simulink model "EcoSIM3_P2_C2_WIP"  (R2014b)
settings: Solver=ode1  SolverMode=SingleTasking  StartTime=0.0  StopTime=4  FixedStep=0.01  RelTol=1e-3
PostLoadFcn:
  | %, if any(exist('dsrtsu_mdlpostloadfcn', 'file') == [2, 3, 6]), try dsrtsu_mdlpostloadfcn('Execute', bdroot); catch fprintf('Error in PostLoadFcn (dsrtsu_mdlpostloadfcn) for model "%s":\n %s\n', bdroot, lasterr); end, end,
InitFcn:
  | tic
  | %Startup_EcoSIM
undefined symbols (not defined in the file or in its folder): canChannel, Controls, DriveCycles, Driver, EM_EFF_MAP, EM_PwrLoss_MAP, EngPwr, EngSpd, EngTrq, Glbl, Overwritten_Mode, Plants, Power, sigbuilder_block, Torque, Trialmap, Veh_Dynamics
libraries: simulink x135, canmsglib x113, fl_lib x104, canlib x89, nesl_utility x56, sdl_lib x29, dspsigops x6, dspswit3 x5, dspstat3 x2, commnoisgen2 x1, dspfdesign x1
(part 10 of 21)

== system EcoSIM3_P2_C2_WIP/Supervisory Controller/Supervisory_IO/VNT Vector/Electrical Rx ==
  Bus Creator : BusCreator  Inputs=7
  Bus Creator{1,4..6,9} (5 alike) : BusCreator  Inputs=2
  Bus Creator2 : BusCreator  Inputs=1
  Bus Creator3 : BusCreator  Inputs=7
  Bus Creator7 : BusCreator  Inputs=1
  Bus Selector : BusSelector  OutputSignals=From_SoftECU.GM_Electrical_Out.Drive_Mode,From_SoftECU.GM_Electrical_Out.PRNDL,From_SoftECU.GM_Electrical_Out.Alpha_Low,From_SoftECU.GM_Electrical_Out.Alpha_High,From_SoftECU.GM_Electrical_Out.Accessory_Wake,From_SoftECU.GM_Electrical_Out.PRNDL_1,From_SoftECU.GM_Electrical_Out.PRNDL_2,From_SoftECU.ESS_Electrical_Out.chga_ena
  Ground{,1..8} (9 alike) : Ground
  Electrical_Rx : Outport
  wires:
  [VNT_Electrical_FromGCM] -> Bus Creator1/1
  [VNT_Electrical_From_SoftECU] -> Bus Creator1/2  "From_SoftECU"
  Bus Creator1/1 -> Bus Selector/1
  Bus Selector/1 -> Bus Creator/1  "<Drive_Mode>"
  Bus Selector/2 -> Bus Creator/2  "<PRNDL>"
  Bus Selector/3 -> Bus Creator/3  "<Alpha_Low>"
  Bus Selector/4 -> Bus Creator/4  "<Alpha_High>"
  Bus Selector/5 -> Bus Creator/5  "<Accessory_Wake>"
  Bus Selector/8 -> Bus Creator2/1  "<chga_ena>"
  Bus Creator/1 -> Bus Creator3/3  "GM_Electrical_Out"
  Bus Creator2/1 -> Bus Creator3/4  "ESS_Electrical_Out"
  Bus Creator3/1 -> Electrical_Rx/1  "Electrical_Rx"
  Ground/1 -> Bus Creator4/1  "Dummy1"
  Ground1/1 -> Bus Creator4/2  "Dummy2"
  Bus Creator4/1 -> Bus Creator3/5  "BAS_Electrical_Out"
  Ground3/1 -> Bus Creator5/2  "Dummy2"
  Ground2/1 -> Bus Creator5/1  "Dummy1"
  Bus Creator5/1 -> Bus Creator3/2  "Clutch_Transmission_Electrical_Out"
  Ground5/1 -> Bus Creator6/2  "Dummy2"
  Ground4/1 -> Bus Creator6/1  "Dummy1"
  Bus Creator6/1 -> Bus Creator3/6  "ICE_Electrical_Out"
  Ground7/1 -> Bus Creator9/2  "Dummy2"
  Ground6/1 -> Bus Creator9/1  "Dummy1"
  Bus Creator9/1 -> Bus Creator3/1  "EM_Electrical_Out"
  Ground8/1 -> Bus Creator7/1  "<Dummy_Electrical1>"
  Bus Creator7/1 -> Bus Creator3/7  "CP1_Electrical_Out"
  Bus Selector/6 -> Bus Creator/6  "<PRNDL_1>"
  Bus Selector/7 -> Bus Creator/7  "<PRNDL_2>"

== system EcoSIM3_P2_C2_WIP/Supervisory Controller/Supervisory_IO/VNT Vector/Electrical Tx ==
  Electrical Tx : Inport
  Bus Creator : BusCreator  Inputs=2
  Bus Selector : BusSelector  OutputSignals=PON,chga_wake
  tag scope: VNT_Electrical_FromMABx=global
  wires:
  Bus Creator/1 -> [VNT_Electrical_FromMABx]  "Supervisory_Electrical_Out"
  Bus Selector/2 -> Bus Creator/2  "<chga_wake>"
  Bus Selector/1 -> Bus Creator/1  "<PON>"
  Electrical Tx/1 -> Bus Selector/1

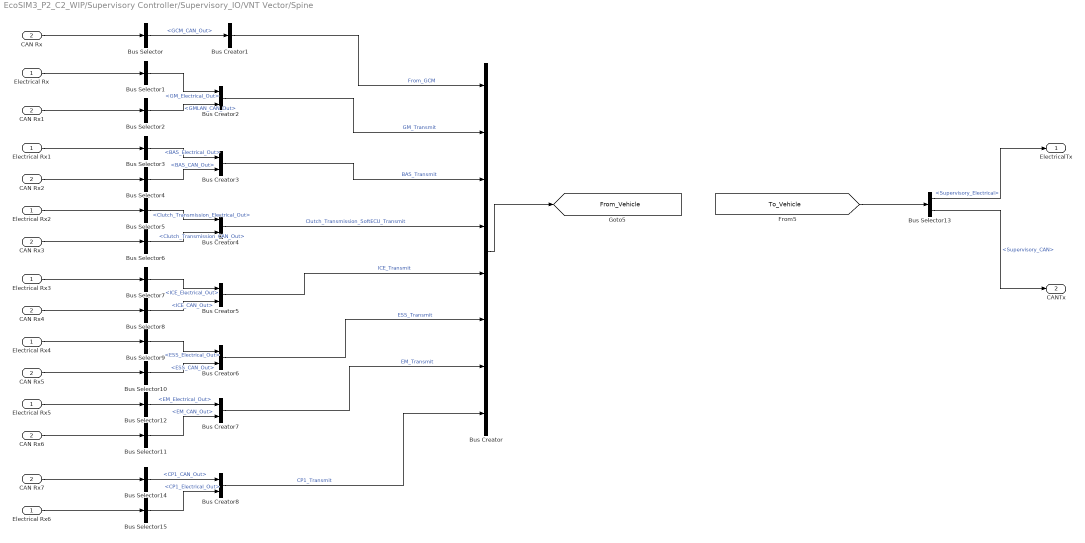
== system EcoSIM3_P2_C2_WIP/Supervisory Controller/Supervisory_IO/VNT Vector/Spine ==
  Electrical Rx : Inport
  CAN Rx : Inport  Port=2
  Bus Creator : BusCreator  Inputs=8
  Bus Creator1 : BusCreator  Inputs=1
  Bus Creator{2..8} (7 alike) : BusCreator  Inputs=2
  Bus Selector : BusSelector  OutputSignals=GCM_CAN_Out
  Bus Selector1 : BusSelector  OutputSignals=GM_Electrical_Out
  Bus Selector10 : BusSelector  OutputSignals=ESS_CAN_Out
  Bus Selector11 : BusSelector  OutputSignals=EM_CAN_Out
  Bus Selector12 : BusSelector  OutputSignals=EM_Electrical_Out
  Bus Selector13 : BusSelector  OutputSignals=Supervisory_Electrical,Supervisory_CAN
  Bus Selector14 : BusSelector  OutputSignals=CP1_CAN_Out
  Bus Selector15 : BusSelector  OutputSignals=CP1_Electrical_Out
  Bus Selector2 : BusSelector  OutputSignals=GMLAN_CAN_Out
  Bus Selector3 : BusSelector  OutputSignals=BAS_Electrical_Out
  Bus Selector4 : BusSelector  OutputSignals=BAS_CAN_Out
  Bus Selector5 : BusSelector  OutputSignals=Clutch_Transmission_Electrical_Out
  Bus Selector6 : BusSelector  OutputSignals=Clutch_Transmission_CAN_Out
  Bus Selector7 : BusSelector  OutputSignals=ICE_Electrical_Out
  Bus Selector8 : BusSelector  OutputSignals=ICE_CAN_Out
  Bus Selector9 : BusSelector  OutputSignals=ESS_Electrical_Out
  CAN Rx{1..7} (7 alike) : InportShadow  Port=2
  Electrical Rx{1..6} (6 alike) : InportShadow
  ElectricalTx : Outport
  CANTx : Outport  Port=2
  tag scope: From_Vehicle=global
  wires:
  [To_Vehicle] -> Bus Selector13/1
  Bus Creator/1 -> [From_Vehicle]
  CAN Rx/1 -> Bus Selector/1
  Electrical Rx/1 -> Bus Selector1/1
  Bus Selector/1 -> Bus Creator1/1  "<GCM_CAN_Out>"
  Bus Creator1/1 -> Bus Creator/1  "From_GCM"
  CAN Rx1/1 -> Bus Selector2/1
  Bus Selector1/1 -> Bus Creator2/1  "<GM_Electrical_Out>"
  Bus Selector2/1 -> Bus Creator2/2  "<GMLAN_CAN_Out>"
  Bus Creator2/1 -> Bus Creator/2  "GM_Transmit"
  Electrical Rx1/1 -> Bus Selector3/1
  CAN Rx2/1 -> Bus Selector4/1
  Bus Selector3/1 -> Bus Creator3/1  "<BAS_Electrical_Out>"
  Bus Selector4/1 -> Bus Creator3/2  "<BAS_CAN_Out>"
  Bus Creator3/1 -> Bus Creator/3  "BAS_Transmit"
  Electrical Rx2/1 -> Bus Selector5/1
  CAN Rx3/1 -> Bus Selector6/1
  Bus Selector5/1 -> Bus Creator4/1  "<Clutch_Transmission_Electrical_Out>"
  Bus Selector6/1 -> Bus Creator4/2  "<Clutch_Transmission_CAN_Out>"
  Bus Creator4/1 -> Bus Creator/4  "Clutch_Transmission_SoftECU_Transmit"
  Electrical Rx3/1 -> Bus Selector7/1
  CAN Rx4/1 -> Bus Selector8/1
  Bus Selector7/1 -> Bus Creator5/1  "<ICE_Electrical_Out>"
  Bus Selector8/1 -> Bus Creator5/2  "<ICE_CAN_Out>"
  Bus Creator5/1 -> Bus Creator/5  "ICE_Transmit"
  Electrical Rx4/1 -> Bus Selector9/1
  CAN Rx5/1 -> Bus Selector10/1
  Bus Selector9/1 -> Bus Creator6/1  "<ESS_Electrical_Out>"
  Bus Selector10/1 -> Bus Creator6/2  "<ESS_CAN_Out>"
  Bus Creator6/1 -> Bus Creator/6  "ESS_Transmit"
  Electrical Rx5/1 -> Bus Selector12/1
  CAN Rx6/1 -> Bus Selector11/1
  Bus Selector12/1 -> Bus Creator7/1  "<EM_Electrical_Out>"
  Bus Selector11/1 -> Bus Creator7/2  "<EM_CAN_Out>"
  Bus Creator7/1 -> Bus Creator/7  "EM_Transmit"
  Bus Selector13/1 -> ElectricalTx/1  "<Supervisory_Electrical>"
  Bus Selector13/2 -> CANTx/1  "<Supervisory_CAN>"
  CAN Rx7/1 -> Bus Selector14/1
  Electrical Rx6/1 -> Bus Selector15/1
  Bus Selector14/1 -> Bus Creator8/1  "<CP1_CAN_Out>"
  Bus Selector15/1 -> Bus Creator8/2  "<CP1_Electrical_Out>"
  Bus Creator8/1 -> Bus Creator/8  "CP1_Transmit"

== system EcoSIM3_P2_C2_WIP/Powertrain/Accessories Power Module/Component Power/The Corrupter/Enabled Subsystem ==
  In1 : Inport
  In2 : Inport  Port=2
  Enable : EnablePort
  Integrator : Integrator  InitialCondition=100
  Product5 : Product  Inputs=*/  RndMeth=Zero
  Out1 : Outport
  wires:
  Integrator/1 -> Out1/1
  In2/1 -> Product5/2
  In1/1 -> Product5/1
  Product5/1 -> Integrator/1

== system EcoSIM3_P2_C2_WIP/Powertrain/Accessories Power Module/Component Power/The Corrupter/Switch Logic ==
  NonCorrupted : Inport
  Corrupted : Inport  Port=2
  Logic : Inport  Port=3
  Switch : Switch  Criteria=u2 > Threshold
  Signal Out : Outport
  wires:
  Switch/1 -> Signal Out/1
  Logic/1 -> Switch/2
  NonCorrupted/1 -> Switch/3
  Corrupted/1 -> Switch/1

== system EcoSIM3_P2_C2_WIP/Powertrain/Accessories Power Module/Component Power/The Corrupter/Switch Logic1 ==
  F : Inport
  L : Inport  Port=2
  NF : Inport  Port=3
  Switch : Switch  Criteria=u2 ~= 0
  Out1 : Outport
  wires:
  L/1 -> Switch/2
  Switch/1 -> Out1/1
  NF/1 -> Switch/3
  F/1 -> Switch/1

== system EcoSIM3_P2_C2_WIP/Powertrain/BAS Motor/ Compnent Model/Sensors/Sensor lag ==
  i : Inport
  1st Order LPF of 1ms in Discrete Form : DiscreteTransferFcn  Numerator=[0.6321]  Denominator=[1 -0.3679]
  o : Outport
  wires:
  i/1 -> 1st Order LPF of 1ms in Discrete Form/1
  1st Order LPF of 1ms in Discrete Form/1 -> o/1

== system EcoSIM3_P2_C2_WIP/Powertrain/BAS Motor/ Compnent Model/Sensors/Sensor lag1 ==
  i : Inport
  1st Order LPF of 1ms in Discrete Form : DiscreteTransferFcn  Numerator=[0.6321]  Denominator=[1 -0.3679]
  o : Outport
  wires:
  1st Order LPF of 1ms in Discrete Form/1 -> o/1
  i/1 -> 1st Order LPF of 1ms in Discrete Form/1

== system EcoSIM3_P2_C2_WIP/Powertrain/BAS Motor/Soft ECU/Algorithm/EEPROM Parameters ==
  note: Need to change this to reflect max speed of the BAS
  Bus Creator : BusCreator  Inputs=2
  Motor_MaxSpeed : Constant  Value=Plants.ICE.Mdl.Plant.red_line_w*Plants.Belt.GR
  POST_Fault : Constant  Value=0
  EEPROM param : Outport
  wires:
  Motor_MaxSpeed/1 -> Bus Creator/1  "Motor_MaxSpeed"
  Bus Creator/1 -> EEPROM param/1
  POST_Fault/1 -> Bus Creator/2  "POST_Fault"

== system EcoSIM3_P2_C2_WIP/Powertrain/BAS Motor/Soft ECU/Algorithm/Faults ==
  Bus Creator : BusCreator  Inputs=3
  Fault_U : Constant  Value=0
  Fault_V : Constant  Value=0
  Fault_W : Constant  Value=0
  Logical Operator : Logic  Operator=OR  Inputs=3  AllPortsSameDT=off  OutDataTypeStr=boolean
  MotorFault : Outport
  CAN : Outport  Port=2
  wires:
  Fault_V/1 -> Logical Operator/2, Bus Creator/2  "Fault_V"
  Bus Creator/1 -> CAN/1
  Fault_U/1 -> Logical Operator/3, Bus Creator/1  "Fault_U"
  Fault_W/1 -> Logical Operator/1, Bus Creator/3  "Fault_W"
  Logical Operator/1 -> MotorFault/1  "MotorFault"

== system EcoSIM3_P2_C2_WIP/Powertrain/BAS Motor/Soft ECU/Algorithm/Torque Determination ==
  Speed : Inport
  IQ : Inport  Port=2
  Gain : Gain  Gain=9.54929659643
  Gain2 : Gain  Gain=9.54929659643
  Gain3 : Gain  Gain=-1
  Gain4 : Gain  Gain=-1
  Iq Lookup1 : Lookup_n-D  BreakpointsForDimension1=Plants.BAS.Mdl.Plant.Iq_reverse  BreakpointsForDimension2=Plants.BAS.Mdl.Plant.Rpm  Table=Plants.BAS.Mdl.Plant.Torque_Iq_1  InternalRulePriority=Speed  RndMeth=Simplest  InputSameDT=on
  Iq Lookup2 : Lookup_n-D  BreakpointsForDimension1=Plants.BAS.Mdl.Plant.Iq_reverse  BreakpointsForDimension2=Plants.BAS.Mdl.Plant.Rpm  Table=Plants.BAS.Mdl.Plant.Torque_Iq_1  InternalRulePriority=Speed  RndMeth=Simplest  InputSameDT=on
  Switch1 : Switch  Criteria=u2 > Threshold
  Switch2 : Switch  Criteria=u2 > Threshold
  Out1 : Outport
  wires:
  Gain2/1 -> Iq Lookup2/2
  Switch1/1 -> Iq Lookup1/1, Iq Lookup2/1
  Gain3/1 -> Switch1/3
  Iq Lookup2/1 -> Switch2/1
  Gain4/1 -> Switch2/3
  IQ/1 -> Switch1/1, Gain3/1, Switch1/2, Switch2/2
  Switch2/1 -> Out1/1
  Gain/1 -> Iq Lookup1/2
  Iq Lookup1/1 -> Gain4/1
  Speed/1 -> Gain2/1, Gain/1

== system EcoSIM3_P2_C2_WIP/Powertrain/Clutch_Transmission2/Trans_Plant/Plant/Gear1-2 ==
  In1 : Inport
  Bus Creator : BusCreator  Inputs=3
  Double-Sided Synchronizer : sdl_lib/Clutches/Double-Sided Synchronizer  model=1  max_torque=1000 N*m  n_teeth=6  clutch_backlash=10 deg  radius=200 mm  clutch_stiffness=1e+7 N*m/rad  clutch_damping=100 N*m/(rad/s)  fric_coeff=0.05  engagement_speed=Inf rad/s  d_o=150 mm  d_i=100 mm  theta=12 deg  friction_model=1  mu_coulomb=0.7  mu_w_vector=[ 0 0.1 0.2 0.3 0.4 0.5 1 2 5 10 100 1000 ] rad/s  mu_coulomb_vector=[ 0.29 0.28 0.26 0.22 0.21 0.2 0.2 0.19 0.19 0.19 0.19 0.19 ]  mu_interp_method=1  mu_extrap_method=1  mu_static=0.9  w_tol=0.001 rad/s  force_min=1 N  peak_force=3 N  width=3 mm  detent_visc_fric_transl=0.1 N/(m/s)  friction_ratio=0.01  v_thr=0.05 m/s  dog_clutch_ring_hub_gap=5 mm  engagement_overlap=3 mm  tooth_height=10 mm  cone_clutch_ring_hub_gap=3 mm  dog_clutch_transl_stiffness=1e+6 N/m  cone_clutch_transl_stiffness=1e+6 N/m  dog_clutch_transl_damping=1000 N/(m/s)  cone_clutch_transl_damping=1000 N/(m/s)  dog_clutch_visc_fric_transl=100 N/(m/s)  initial_state_locked=3  dog_clutch_init_pos=0 mm  cone_clutch_init_pos=0 mm  init_rel_angle_A=0 deg  init_rel_angle_B=0 deg
  Gain : Gain  Gain=1000
  Gain1 : Gain  Gain=1000
  Ideal Force Source : fl_lib/Mechanical/Mechanical Sources/Ideal Force Source
  Mechanical Translational Reference : fl_lib/Mechanical/Translational Elements/Mechanical Translational Reference
  Memory : Memory
  PI : Subsystem
  PS-Simulink Converter : nesl_utility/PS-Simulink Converter  PhysicalDomain=network_engine_domain  SubClassName=ps_output  LeftPortType=input  RightPortType=output  PseudoPeriodic=off  Frequencies=[]  Unit=1  AffineConversion=off
  PS-Simulink Converter1 : nesl_utility/PS-Simulink Converter  PhysicalDomain=network_engine_domain  SubClassName=ps_output  LeftPortType=input  RightPortType=output  PseudoPeriodic=off  Frequencies=[]  Unit=1  AffineConversion=off
  Rate Transition2 : RateTransition
  Scope7 : Scope
      settings: SaveName=ScopeData7
  Shaft Position : Subsystem
  Shift linkage mass : fl_lib/Mechanical/Translational Elements/Mass  mass=1 kg  v_specify=on  v_priority=High  v=0 m/s  f_specify=off  f_priority=High  f=0 N
  Simple Gear : sdl_lib/Gears/Simple Gear  ratio=Plants.Trans.Mdl.Plant.GR(1)  rotation_direction=1  friction_model=1  T_noload=0.1 N*m  T_nom=5 N*m  efficiency_nom=0.8  efficiency=0.8  mu_visc=[ 0 0 ] N*m/(rad/s)  w_thr=0.01 rad/s
  Simple Gear1 : sdl_lib/Gears/Simple Gear  ratio=Plants.Trans.Mdl.Plant.GR(2)  rotation_direction=1  friction_model=1  T_noload=0.1 N*m  T_nom=5 N*m  efficiency_nom=0.8  efficiency=0.8  mu_visc=[ 0 0 ] N*m/(rad/s)  w_thr=0.01 rad/s
  Simulink-PS Converter : nesl_utility/Simulink-PS Converter  PhysicalDomain=network_engine_domain  SubClassName=ps_input  LeftPortType=input  RightPortType=output  PseudoPeriodic=off  Frequencies=[]  NoiseDistribution=none  NoiseParameters=[]  Unit=N  AffineConversion=off  InputFiltering=on  SimscapeFilterOrder=1  InputFilterTimeConstant=0.01  UdotUserProvided=1
  Out : PMIOPort  Port=1  Side=Right
  In : PMIOPort  Port=2  Side=Left
  ShaftPosn : Outport
  wires:
  Rate Transition2/1 -> Simulink-PS Converter/1, Scope7/1
  PI/1(Force) -> Rate Transition2/1
  PS-Simulink Converter/1 -> Gain/1
  PS-Simulink Converter1/1 -> Gain1/1
  Gain/1 -> Memory/1, Shaft Position/1(Position_mm), Bus Creator/2  "Shaft_1-2_Dog_Clutch_posn_mm"
  Memory/1 -> PI/1(Actual_Pos)
  Gain1/1 -> Bus Creator/3  "Shaft_1-2_Cone_Clutch_posn_mm"
  In1/1 -> PI/2(Desired_Pos)
  Bus Creator/1 -> ShaftPosn/1  "Shaft_1-2"
  Shaft Position/1(Position) -> Bus Creator/1  "Shaft_1-2_Position"
  connections:
  Ideal Force Source/LConn1 -- Double-Sided Synchronizer/LConn1 -- Shift linkage mass/LConn1
  Ideal Force Source/RConn2 -- Mechanical Translational Reference/LConn1
  Ideal Force Source/RConn1 -- Simulink-PS Converter/RConn1
  Double-Sided Synchronizer/LConn3 -- Simple Gear/RConn1
  Double-Sided Synchronizer/RConn3 -- Simple Gear1/RConn1
  PS-Simulink Converter/LConn1 -- Double-Sided Synchronizer/RConn1
  Double-Sided Synchronizer/RConn2 -- PS-Simulink Converter1/LConn1
  Out/RConn1 -- Double-Sided Synchronizer/LConn2
  In/RConn1 -- Simple Gear/LConn1 -- Simple Gear1/LConn1

== system EcoSIM3_P2_C2_WIP/Powertrain/Clutch_Transmission2/Trans_Plant/Plant/Gear3-4 ==
  In1 : Inport
  Bus Creator : BusCreator  Inputs=3
  Double-Sided Synchronizer : sdl_lib/Clutches/Double-Sided Synchronizer  model=1  max_torque=1000 N*m  n_teeth=6  clutch_backlash=10 deg  radius=200 mm  clutch_stiffness=1e+7 N*m/rad  clutch_damping=100 N*m/(rad/s)  fric_coeff=0.05  engagement_speed=Inf rad/s  d_o=150 mm  d_i=100 mm  theta=12 deg  friction_model=1  mu_coulomb=0.7  mu_w_vector=[ 0 0.1 0.2 0.3 0.4 0.5 1 2 5 10 100 1000 ] rad/s  mu_coulomb_vector=[ 0.29 0.28 0.26 0.22 0.21 0.2 0.2 0.19 0.19 0.19 0.19 0.19 ]  mu_interp_method=1  mu_extrap_method=1  mu_static=0.9  w_tol=0.001 rad/s  force_min=1 N  peak_force=3 N  width=3 mm  detent_visc_fric_transl=0.1 N/(m/s)  friction_ratio=0.01  v_thr=0.05 m/s  dog_clutch_ring_hub_gap=5 mm  engagement_overlap=3 mm  tooth_height=10 mm  cone_clutch_ring_hub_gap=3 mm  dog_clutch_transl_stiffness=1e+6 N/m  cone_clutch_transl_stiffness=1e+6 N/m  dog_clutch_transl_damping=1000 N/(m/s)  cone_clutch_transl_damping=1000 N/(m/s)  dog_clutch_visc_fric_transl=100 N/(m/s)  initial_state_locked=3  dog_clutch_init_pos=0 mm  cone_clutch_init_pos=0 mm  init_rel_angle_A=0 deg  init_rel_angle_B=0 deg
  Gain : Gain  Gain=1000
  Gain1 : Gain  Gain=1000
  Ideal Force Source : fl_lib/Mechanical/Mechanical Sources/Ideal Force Source
  Mechanical Translational Reference : fl_lib/Mechanical/Translational Elements/Mechanical Translational Reference
  Memory : Memory
  PI2 : Subsystem
  PS-Simulink Converter : nesl_utility/PS-Simulink Converter  PhysicalDomain=network_engine_domain  SubClassName=ps_output  LeftPortType=input  RightPortType=output  PseudoPeriodic=off  Frequencies=[]  Unit=1  AffineConversion=off
  PS-Simulink Converter1 : nesl_utility/PS-Simulink Converter  PhysicalDomain=network_engine_domain  SubClassName=ps_output  LeftPortType=input  RightPortType=output  PseudoPeriodic=off  Frequencies=[]  Unit=1  AffineConversion=off
  Rate Transition2 : RateTransition
  Scope7 : Scope
      settings: SaveName=ScopeData7
  Shaft Position : Subsystem
  Shift linkage mass : fl_lib/Mechanical/Translational Elements/Mass  mass=1 kg  v_specify=on  v_priority=High  v=0 m/s  f_specify=off  f_priority=High  f=0 N
  Simple Gear2 : sdl_lib/Gears/Simple Gear  ratio=Plants.Trans.Mdl.Plant.GR(3)  rotation_direction=1  friction_model=1  T_noload=0.1 N*m  T_nom=5 N*m  efficiency_nom=0.8  efficiency=0.8  mu_visc=[ 0 0 ] N*m/(rad/s)  w_thr=0.01 rad/s
  Simple Gear3 : sdl_lib/Gears/Simple Gear  ratio=Plants.Trans.Mdl.Plant.GR(4)  rotation_direction=1  friction_model=1  T_noload=0.1 N*m  T_nom=5 N*m  efficiency_nom=0.8  efficiency=0.8  mu_visc=[ 0 0 ] N*m/(rad/s)  w_thr=0.01 rad/s
  Simulink-PS Converter : nesl_utility/Simulink-PS Converter  PhysicalDomain=network_engine_domain  SubClassName=ps_input  LeftPortType=input  RightPortType=output  PseudoPeriodic=off  Frequencies=[]  NoiseDistribution=none  NoiseParameters=[]  Unit=N  AffineConversion=off  InputFiltering=on  SimscapeFilterOrder=1  InputFilterTimeConstant=0.01  UdotUserProvided=1
  Out : PMIOPort  Port=1  Side=Right
  In : PMIOPort  Port=2  Side=Left
  ShaftPosn : Outport
  wires:
  Gain1/1 -> Bus Creator/3  "Shaft_3-4_Cone_Clutch_posn_mm"
  Gain/1 -> Bus Creator/2, Memory/1, Shaft Position/1(Position_mm)  "Shaft_3-4_Dog_Clutch_posn_mm"
  PS-Simulink Converter1/1 -> Gain1/1
  PS-Simulink Converter/1 -> Gain/1
  PI2/1(Force) -> Rate Transition2/1
  Rate Transition2/1 -> Scope7/1, Simulink-PS Converter/1
  Bus Creator/1 -> ShaftPosn/1  "Shaft_3-4"
  Memory/1 -> PI2/1(Actual_Pos)
  In1/1 -> PI2/2(Desired_Pos)
  Shaft Position/1(Position) -> Bus Creator/1  "Shaft_3-4_Position"
  connections:
  Out/RConn1 -- Double-Sided Synchronizer/LConn2
  Double-Sided Synchronizer/RConn2 -- PS-Simulink Converter1/LConn1
  PS-Simulink Converter/LConn1 -- Double-Sided Synchronizer/RConn1
  Simple Gear3/RConn1 -- Double-Sided Synchronizer/RConn3
  Simple Gear2/RConn1 -- Double-Sided Synchronizer/LConn3
  Ideal Force Source/RConn1 -- Simulink-PS Converter/RConn1
  Ideal Force Source/RConn2 -- Mechanical Translational Reference/LConn1
  Double-Sided Synchronizer/LConn1 -- Shift linkage mass/LConn1 -- Ideal Force Source/LConn1
  Simple Gear2/LConn1 -- In/RConn1 -- Simple Gear3/LConn1

== system EcoSIM3_P2_C2_WIP/Powertrain/Clutch_Transmission2/Trans_Plant/Plant/Gear5-R ==
  In1 : Inport
  Bus Creator : BusCreator  Inputs=3
  Double-Sided Synchronizer : sdl_lib/Clutches/Double-Sided Synchronizer  model=1  max_torque=1000 N*m  n_teeth=6  clutch_backlash=10 deg  radius=200 mm  clutch_stiffness=1e+7 N*m/rad  clutch_damping=100 N*m/(rad/s)  fric_coeff=0.05  engagement_speed=Inf rad/s  d_o=150 mm  d_i=100 mm  theta=12 deg  friction_model=1  mu_coulomb=0.7  mu_w_vector=[ 0 0.1 0.2 0.3 0.4 0.5 1 2 5 10 100 1000 ] rad/s  mu_coulomb_vector=[ 0.29 0.28 0.26 0.22 0.21 0.2 0.2 0.19 0.19 0.19 0.19 0.19 ]  mu_interp_method=1  mu_extrap_method=1  mu_static=0.9  w_tol=0.001 rad/s  force_min=1 N  peak_force=3 N  width=3 mm  detent_visc_fric_transl=0.1 N/(m/s)  friction_ratio=0.01  v_thr=0.05 m/s  dog_clutch_ring_hub_gap=5 mm  engagement_overlap=3 mm  tooth_height=10 mm  cone_clutch_ring_hub_gap=3 mm  dog_clutch_transl_stiffness=1e+6 N/m  cone_clutch_transl_stiffness=1e+6 N/m  dog_clutch_transl_damping=1000 N/(m/s)  cone_clutch_transl_damping=1000 N/(m/s)  dog_clutch_visc_fric_transl=100 N/(m/s)  initial_state_locked=3  dog_clutch_init_pos=0 mm  cone_clutch_init_pos=0 mm  init_rel_angle_A=0 deg  init_rel_angle_B=0 deg
  Gain : Gain  Gain=1000
  Gain1 : Gain  Gain=1000
  Ideal Force Source : fl_lib/Mechanical/Mechanical Sources/Ideal Force Source
  Mechanical Translational Reference : fl_lib/Mechanical/Translational Elements/Mechanical Translational Reference
  Memory : Memory
  PI2 : Subsystem
  PS-Simulink Converter : nesl_utility/PS-Simulink Converter  PhysicalDomain=network_engine_domain  SubClassName=ps_output  LeftPortType=input  RightPortType=output  PseudoPeriodic=off  Frequencies=[]  Unit=1  AffineConversion=off
  PS-Simulink Converter1 : nesl_utility/PS-Simulink Converter  PhysicalDomain=network_engine_domain  SubClassName=ps_output  LeftPortType=input  RightPortType=output  PseudoPeriodic=off  Frequencies=[]  Unit=1  AffineConversion=off
  Rate Transition2 : RateTransition
  Scope7 : Scope
      settings: SaveName=ScopeData7
  Shaft Position : Subsystem
  Shift linkage mass : fl_lib/Mechanical/Translational Elements/Mass  mass=1 kg  v_specify=on  v_priority=High  v=0 m/s  f_specify=off  f_priority=High  f=0 N
  Simple Gear2 : sdl_lib/Gears/Simple Gear  ratio=Plants.Trans.Mdl.Plant.GR(5)  rotation_direction=1  friction_model=1  T_noload=0.1 N*m  T_nom=5 N*m  efficiency_nom=0.8  efficiency=0.8  mu_visc=[ 0 0 ] N*m/(rad/s)  w_thr=0.01 rad/s
  Simple Gear3 : sdl_lib/Gears/Simple Gear  ratio=2.76  rotation_direction=2  friction_model=1  T_noload=0.1 N*m  T_nom=5 N*m  efficiency_nom=0.8  efficiency=0.8  mu_visc=[ 0 0 ] N*m/(rad/s)  w_thr=0.01 rad/s
  Simulink-PS Converter : nesl_utility/Simulink-PS Converter  PhysicalDomain=network_engine_domain  SubClassName=ps_input  LeftPortType=input  RightPortType=output  PseudoPeriodic=off  Frequencies=[]  NoiseDistribution=none  NoiseParameters=[]  Unit=N  AffineConversion=off  InputFiltering=on  SimscapeFilterOrder=1  InputFilterTimeConstant=0.01  UdotUserProvided=1
  Out : PMIOPort  Port=1  Side=Right
  In : PMIOPort  Port=2  Side=Left
  ShaftPosn : Outport
  wires:
  In1/1 -> PI2/2(Desired_Pos)
  Memory/1 -> PI2/1(Actual_Pos)
  Bus Creator/1 -> ShaftPosn/1  "Shaft_5-R"
  Rate Transition2/1 -> Simulink-PS Converter/1, Scope7/1
  PI2/1(Force) -> Rate Transition2/1
  PS-Simulink Converter/1 -> Gain/1
  PS-Simulink Converter1/1 -> Gain1/1
  Gain/1 -> Bus Creator/2, Memory/1, Shaft Position/1(Position_mm)  "Shaft_5-R_Dog_Clutch_posn_mm"
  Gain1/1 -> Bus Creator/3  "Shaft_5-R_Cone_Clutch_posn_mm"
  Shaft Position/1(Position) -> Bus Creator/1  "Shaft_5-R_Position"
  connections:
  In/RConn1 -- Simple Gear2/LConn1 -- Simple Gear3/LConn1
  Ideal Force Source/LConn1 -- Shift linkage mass/LConn1 -- Double-Sided Synchronizer/LConn1
  Ideal Force Source/RConn2 -- Mechanical Translational Reference/LConn1
  Ideal Force Source/RConn1 -- Simulink-PS Converter/RConn1
  Simple Gear2/RConn1 -- Double-Sided Synchronizer/LConn3
  Simple Gear3/RConn1 -- Double-Sided Synchronizer/RConn3
  PS-Simulink Converter/LConn1 -- Double-Sided Synchronizer/RConn1
  Double-Sided Synchronizer/RConn2 -- PS-Simulink Converter1/LConn1
  Out/RConn1 -- Double-Sided Synchronizer/LConn2

== system EcoSIM3_P2_C2_WIP/Powertrain/Clutch_Transmission2/Trans_Plant/Plant/Subsystem ==
  In1 : Inport
  Bus Selector : BusSelector  OutputSignals=Shaft_1-2.Shaft_1-2_Position,Shaft_3-4.Shaft_3-4_Position,Shaft_5-R.Shaft_5-R_Position
  Determine Gear : Stateflow chart  Commented=on  TreatAsAtomicUnit=on
  Display : Display
  Gain : Gain
  Lookup Table based Gear : Subsystem  Commented=on
  Memory : Memory
  Mux : Mux  Inputs=3
  Scope : Scope
      settings: SaveName=ScopeData3
  Switch : Switch  Criteria=u2 > Threshold  Threshold=6
  Truth Table : Truth Table  TreatAsAtomicUnit=on
  Out1 : Outport
  tag scope: Shaft_Positions=global
  wires:
  In1/1 -> Bus Selector/1
  Bus Selector/3 -> Truth Table/3(u3), Mux/3  "<Shaft_5-R_Position>"
  Bus Selector/2 -> Truth Table/2(u2), Mux/2  "<Shaft_3-4_Position>"
  Bus Selector/1 -> Truth Table/1(u1), Mux/1  "<Shaft_1-2_Position>"
  Switch/1 -> Memory/1, Gain/1  "Mastershift_Gear"
  Gain/1 -> Display/1, Out1/1
  Mux/1 -> [Shaft_Positions], Scope/1
  Truth Table/1(y) -> Switch/3, Switch/2  "Mastershift_Gear"
  Memory/1 -> Switch/1

== system EcoSIM3_P2_C2_WIP/Powertrain/Electric Motor / Component Model/Plant/EM_Thermal_Model ==
  note: Instead of a heat source, add convection to the water
  note: A hotspot that will be the thermally weakest point
  note: Assume coolant out temp is same as motor temp
  EM_Power_Loss : Inport
  Conductive Heat Transfer : fl_lib/Thermal/Thermal Elements/Conductive Heat Transfer  area=4 cm^2  thickness=0.1 cm  th_cond=401 W/(m*K)  Q_specify=off  Q_priority=High  Q=0 J/s  T_specify=off  T_priority=High  T=0 K
  Constant1 : Constant  Value=293
  Convection to air : fl_lib/Thermal/Thermal Elements/Convective Heat Transfer  area=1111 cm^2  heat_tr_coeff=10 W/(m^2 * K)  Q_specify=off  Q_priority=High  Q=0 J/s  T_specify=off  T_priority=High  T=0 K
  EM_Over_Temp_Fault : Subsystem
  Gain : Gain  Gain=0.05
  Gain1 : Gain  Gain=0.95
  Heat Dissipated through coolant : Subsystem
  Heat absorbed by coolant : fl_lib/Thermal/Thermal Sources/Ideal Heat Flow Source
  Hotspot Heat : fl_lib/Thermal/Thermal Sources/Ideal Heat Flow Source
  Hotspot Thermal mass : fl_lib/Thermal/Thermal Elements/Thermal Mass  mass=0.1 kg  sp_heat=447 J/kg/K  Q_specify=off  Q_priority=High  Q=0 J/s  T_specify=off  T_priority=High  T=300 K
  Hotspot temp in °C : Scope
      settings: SaveName=ScopeData2
  Ideal Temperature Source : fl_lib/Thermal/Thermal Sources/Ideal Temperature Source
  Memory : Memory  X0=293
  Memory1 : Memory  X0=25
  Motor Heat Loss : fl_lib/Thermal/Thermal Sources/Ideal Heat Flow Source
  Motor Thermal Mass : fl_lib/Thermal/Thermal Elements/Thermal Mass  mass=35 kg  sp_heat=447 J/kg/K  Q_specify=off  Q_priority=High  Q=0 J/s  T_specify=off  T_priority=High  T=300 K
  Simulink-PS Converter : nesl_utility/Simulink-PS Converter  PhysicalDomain=network_engine_domain  SubClassName=ps_input  LeftPortType=input  RightPortType=output  PseudoPeriodic=off  Frequencies=[]  NoiseDistribution=none  NoiseParameters=[]  Unit=J/s  AffineConversion=off  InputFiltering=off  SimscapeFilterOrder=1  InputFilterTimeConstant=0.001  UdotUserProvided=1
  Simulink-PS Converter1 : nesl_utility/Simulink-PS Converter  PhysicalDomain=network_engine_domain  SubClassName=ps_input  LeftPortType=input  RightPortType=output  PseudoPeriodic=off  Frequencies=[]  NoiseDistribution=none  NoiseParameters=[]  Unit=J/s  AffineConversion=off  InputFiltering=off  SimscapeFilterOrder=1  InputFilterTimeConstant=0.001  UdotUserProvided=1
  Simulink-PS Converter2 : nesl_utility/Simulink-PS Converter  PhysicalDomain=network_engine_domain  SubClassName=ps_input  LeftPortType=input  RightPortType=output  PseudoPeriodic=off  Frequencies=[]  NoiseDistribution=none  NoiseParameters=[]  Unit=K  AffineConversion=off  InputFiltering=off  SimscapeFilterOrder=1  InputFilterTimeConstant=0.001  UdotUserProvided=1
  Solver Configuration : nesl_utility/Solver Configuration  PhysicalDomain=network_engine_domain  SubClassName=solver  LeftPortType=input  RightPortType=generic  Accelerate=off  Tones=[]  Harmonics=[]  SimulateNoise=off  Profile=off  UseLocalSampling=off  EnableSwitchedLinearOptims=on  FrequencyDomain=off  UseCCode=off  RelTol=0.001  AbsTol=1e-06  MinStep=1e-09  ToWorkspace=off  DoDC=off  ResidualTolerance=1e-09  UseLocalSolver=on  LocalSolverChoice=NE_BACKWARD_EULER_ADVANCER  LocalSolverSampleTime=0.01  DoFixedCost=off  MaxNonlinIter=3  MaxModeIter=2  LinearAlgebra=Sparse  DelaysMemoryBudget=1024  AutomaticFiltering=on  FilteringTimeConstant=0.001
  Temp Hotspot : Subsystem
  Temp Motor : Subsystem
  Thermal Reference{,2..4} (4 alike) : fl_lib/Thermal/Thermal Elements/Thermal Reference
  Out1 : Outport
  wires:
  Constant1/1 -> Simulink-PS Converter2/1
  Temp Hotspot/1(Temp C) -> Hotspot temp in °C/1  "EM_hotspot_Temperature_degC"
  Temp Motor/1(Temp K) -> Memory/1
  EM_Over_Temp_Fault/1(Out1) -> Out1/1  "EM_Temperature_degC"
  Memory/1 -> Heat Dissipated through coolant/1(Coolant Out Temp)
  EM_Power_Loss/1 -> Gain/1, Gain1/1  "EM_Power_loss_W"
  Gain/1 -> Simulink-PS Converter/1
  Gain1/1 -> Simulink-PS Converter1/1
  Temp Motor/2(Temp C) -> Memory1/1  "EM_Temperature_degC"
  Memory1/1 -> EM_Over_Temp_Fault/1(In1)  "EM_Temperature_degC"
  connections:
  Simulink-PS Converter2/RConn1 -- Ideal Temperature Source/RConn1
  Heat Dissipated through coolant/RConn1 -- Heat absorbed by coolant/RConn1
  Convection to air/RConn1 -- Ideal Temperature Source/LConn1
  Thermal Reference4/LConn1 -- Hotspot Heat/RConn2
  Simulink-PS Converter1/RConn1 -- Hotspot Heat/RConn1
  Thermal Reference/LConn1 -- Motor Heat Loss/RConn2
  Thermal Reference2/LConn1 -- Ideal Temperature Source/RConn2
  Thermal Reference3/LConn1 -- Heat absorbed by coolant/RConn2
  Motor Heat Loss/RConn1 -- Simulink-PS Converter/RConn1 -- Solver Configuration/RConn1
  Convection to air/LConn1 -- Temp Motor/LConn1 -- Conductive Heat Transfer/RConn1 -- Motor Thermal Mass/LConn1 -- Heat absorbed by coolant/LConn1 -- Motor Heat Loss/LConn1
  Conductive Heat Transfer/LConn1 -- Hotspot Thermal mass/LConn1 -- Temp Hotspot/LConn1 -- Hotspot Heat/LConn1

== system EcoSIM3_P2_C2_WIP/Powertrain/Electric Motor / Component Model/Sensors/Fault Insertation ==
  In1 : Inport
  Additional_Torque_Nm_Default : Constant  Value=0
  Gain : Gain  Gain=.3
  Ideal Torque Source1 : fl_lib/Mechanical/Mechanical Sources/Ideal Torque Source
  Mechanical Rotational Reference2 : fl_lib/Mechanical/Rotational Elements/Mechanical Rotational Reference
  OverTorque_Trigger : Switch  Criteria=u2 > Threshold  Threshold=0.5
  Simulink-PS Converter1 : nesl_utility/Simulink-PS Converter  PhysicalDomain=network_engine_domain  SubClassName=ps_input  LeftPortType=input  RightPortType=output  PseudoPeriodic=off  Frequencies=[]  NoiseDistribution=none  NoiseParameters=[]  Unit=1  AffineConversion=off  InputFiltering=off  SimscapeFilterOrder=1  InputFilterTimeConstant=0.001  UdotUserProvided=1
  Conn1 : PMIOPort  Port=1  Side=Right
  wires:
  [EM_OverTorque_Trigger] -> OverTorque_Trigger/2
  Additional_Torque_Nm_Default/1 -> OverTorque_Trigger/3
  OverTorque_Trigger/1 -> Simulink-PS Converter1/1
  In1/1 -> Gain/1
  Gain/1 -> OverTorque_Trigger/1
  connections:
  Simulink-PS Converter1/RConn1 -- Ideal Torque Source1/RConn1
  Ideal Torque Source1/RConn2 -- Mechanical Rotational Reference2/LConn1
  Ideal Torque Source1/LConn1 -- Conn1/RConn1

== system EcoSIM3_P2_C2_WIP/Powertrain/Electric Motor / Component Model/Sensors/Sensor lag ==
  i : Inport
  1st Order LPF of 1ms in Discrete Form : DiscreteTransferFcn  Numerator=[0.6321]  Denominator=[1 -0.3679]
  o : Outport
  wires:
  i/1 -> 1st Order LPF of 1ms in Discrete Form/1
  1st Order LPF of 1ms in Discrete Form/1 -> o/1

== system EcoSIM3_P2_C2_WIP/Powertrain/Electric Motor / Component Model/Sensors/Sensor lag1 ==
  i : Inport
  1st Order LPF of 1ms in Discrete Form : DiscreteTransferFcn  Numerator=[0.6321]  Denominator=[1 -0.3679]
  o : Outport
  wires:
  i/1 -> 1st Order LPF of 1ms in Discrete Form/1
  1st Order LPF of 1ms in Discrete Form/1 -> o/1

== system EcoSIM3_P2_C2_WIP/Powertrain/Electric Motor / Component Model/Sensors/Sensors ==
  note: Sensor Model: Place where we add Corrupter
  Bus Creator : BusCreator  Inputs=2
  Ideal Rotational Motion Sensor : fl_lib/Mechanical/Mechanical Sensors/Ideal Rotational Motion Sensor  offset=0 rad
  Ideal Torque Sensor : fl_lib/Mechanical/Mechanical Sensors/Ideal Torque Sensor
  Mechanical Rotational Reference1 : fl_lib/Mechanical/Rotational Elements/Mechanical Rotational Reference
  PS-Simulink Converter : nesl_utility/PS-Simulink Converter  PhysicalDomain=network_engine_domain  SubClassName=ps_output  LeftPortType=input  RightPortType=output  PseudoPeriodic=off  Frequencies=[]  Unit=1  AffineConversion=off
  PS-Simulink Converter1 : nesl_utility/PS-Simulink Converter  PhysicalDomain=network_engine_domain  SubClassName=ps_output  LeftPortType=input  RightPortType=output  PseudoPeriodic=off  Frequencies=[]  Unit=1  AffineConversion=off
  Sensor lag : Subsystem
  Sensor lag1 : Subsystem
  Shaft : PMIOPort  Port=1  Side=Left
  To_Plants : PMIOPort  Port=2  Side=Right
  EM_Shaft_out : Outport
  wires:
  Sensor lag/1(o) -> Bus Creator/1  "EM_Speed_produced_rad_per_s"
  Sensor lag1/1(o) -> Bus Creator/2  "EM_Torque_Produced_Nm"
  Bus Creator/1 -> EM_Shaft_out/1  "EM_Shaft"
  PS-Simulink Converter/1 -> Sensor lag/1(i)  "EM_Speed_produced_rad_per_s"
  PS-Simulink Converter1/1 -> Sensor lag1/1(i)  "EM_Torque_Produced_Nm"
  connections:
  Ideal Torque Sensor/LConn1 -- Shaft/RConn1 -- Ideal Rotational Motion Sensor/LConn1
  Ideal Rotational Motion Sensor/RConn1 -- Mechanical Rotational Reference1/LConn1
  PS-Simulink Converter/LConn1 -- Ideal Rotational Motion Sensor/RConn2
  PS-Simulink Converter1/LConn1 -- Ideal Torque Sensor/RConn2
  Ideal Torque Sensor/RConn1 -- To_Plants/RConn1

== system EcoSIM3_P2_C2_WIP/Powertrain/Electric Motor /Soft ECU/Algorithm/Normal Operation ==
  note: These signals are supposed to be
      |  coming in through CAN
  SignalIn : Inport
  FaultTrigger : Inport  Port=2
  Enable : EnablePort  StatesWhenEnabling=reset
  Bus Creator : BusCreator  Inputs=3
  Bus Selector : BusSelector  OutputSignals=Motor_MaxSpeed
  Bus Selector1 : BusSelector  OutputSignals=EM_Sensors.Motor_Speed,EM_Sensors.InternalMotorError,EM_CAN_Messages.EM_CAN.M192_Command_Message.Rotation_Direction,EM_CAN_Messages.EM_CAN.M192_Command_Message.Torque_Command,ESS_CAN_Out.BCM_Status.bcm_mainc_stat,EM_CAN_Messages.EM_CAN.M192_Command_Message.Inverter_Enable,EM_CAN_Messages.EM_Electrical.EM_Powerup
  Bus Selector4 : BusSelector  OutputSignals=EM_torque_cmd_value,EM_torque_cmd_trigger
  EEPROM Parameters1 : Subsystem
  Normal_Operation : Stateflow chart  TreatAsAtomicUnit=on
  Scope : Scope
      settings: SaveName=ScopeData58
  Switch : Switch  Criteria=u2 > Threshold  Threshold=0.5
  Status : Outport
  wires:
  Bus Selector1/3 -> Normal_Operation/3(Rotation_Direction)  "<Rotation_Direction>"
  Bus Selector1/4 -> Normal_Operation/4(Torque_Command)  "<Torque_Command>"
  SignalIn/1 -> Bus Selector1/1
  Bus Selector/1 -> Normal_Operation/8(Motor_MaxSpeed)  "<Motor_MaxSpeed>"
  Normal_Operation/1(Commanded_Torque) -> Switch/3
  EEPROM Parameters1/1(EEPROM param) -> Bus Selector/1
  Bus Selector1/5 -> Normal_Operation/5(batt_mainc_stat)  "<bcm_mainc_stat>"
  Bus Selector1/6 -> Normal_Operation/6(Inverter_Enable)  "<Inverter_Enable>"
  Switch/1 -> Scope/1, Bus Creator/1  "Commanded_Torque"
  FaultTrigger/1 -> Bus Selector4/1
  Bus Selector4/2 -> Switch/2  "<EM_torque_cmd_trigger>"
  Bus Selector4/1 -> Switch/1  "<EM_torque_cmd_value>"
  Bus Selector1/1 -> Normal_Operation/1(Motor_Speed)  "<Motor_Speed>"
  Bus Selector1/2 -> Normal_Operation/2(InternalMotorError)  "<InternalMotorError>"
  Bus Creator/1 -> Status/1  "RunningStatus"
  Normal_Operation/2(RUN_Fault) -> Bus Creator/2  "RUN_Fault"
  Normal_Operation/3(ShutdownRequest) -> Bus Creator/3  "ShutdownRequest"
  Bus Selector1/7 -> Normal_Operation/7(Power_up)  "<EM_Powerup>"

== system EcoSIM3_P2_C2_WIP/Powertrain/Electric Motor /Soft ECU/Algorithm/Rinehart Documentation ==

== system EcoSIM3_P2_C2_WIP/Powertrain/Electric Motor /Soft ECU/Algorithm/Startup_Shutdown ==
  SignalIn : Inport
  Faults : Inport  Port=2
  Bus Creator : BusCreator  Inputs=7
  Bus Selector : BusSelector  OutputSignals=EM_Sensors.EM_Temperature_degC,EM_Sensors.Motor_Speed,EM_Sensors.EM_Torque_Out_Nm,EM_CAN_Messages.EM_CAN.M192_Command_Message.Rotation_Direction,EM_CAN_Messages.EM_Electrical.EM_Powerup,EM_Sensors.InternalMotorError,ESS_CAN_Out.BCM_Status.bcm_mainc_stat,EM_CAN_Messages.EM_CAN.M192_Command_Message.Inverter_Enable
  Bus Selector1 : BusSelector  OutputSignals=KeySwMode,POST_Fault
  Bus Selector3 : BusSelector  OutputSignals=RUN_Fault,ShutdownRequest
  EEPROM Parameters : Subsystem
  Memory : Memory
  Memory1 : Memory
  Memory2 : Memory
  Startup-Shutdown : Stateflow chart  TreatAsAtomicUnit=on
  Subsystem : Subsystem
  Temperature Values Dummy : Subsystem
  Terminator : Terminator
  Inverter_Status : Outport
  VSM : Outport  Port=2
  wires:
  Startup-Shutdown/2(Inverter_Enable_Lockout) -> Bus Creator/6  "Inverter_Enable_Lockout"
  Bus Selector/6 -> Startup-Shutdown/2(InternalMotorError)  "<InternalMotorError>"
  SignalIn/1 -> Bus Selector/1
  EEPROM Parameters/1(EEPROM param) -> Bus Selector1/1
  Bus Selector1/1 -> Startup-Shutdown/7(KeySwMode)  "<KeySwMode>"
  Bus Selector1/2 -> Startup-Shutdown/8(POST_Fault), Bus Creator/7  "<POST_Fault>"
  Bus Selector/7 -> Startup-Shutdown/3(batt_mainc_stat)  "<bcm_mainc_stat>"
  Bus Selector/8 -> Startup-Shutdown/4(Inverter_Enable)  "<Inverter_Enable>"
  Bus Selector/5 -> Startup-Shutdown/1(Power_up)  "<EM_Powerup>"
  Bus Selector/4 -> Memory1/1  "<Rotation_Direction>"
  Temperature Values Dummy/1(TempValues) -> Bus Creator/1  "Temperatures"
  Bus Selector/1 -> Temperature Values Dummy/1(FromPlant)  "<EM_Temperature_degC>"
  Bus Selector/2 -> Bus Creator/2  "<Motor_Speed>"
  Startup-Shutdown/1(VSM_Mode) -> Subsystem/2(VSM_In)
  Subsystem/1(Dir) -> Bus Creator/4
  Memory1/1 -> Subsystem/1(Dir_In)  "Direction_Feedback"
  Bus Selector/3 -> Bus Creator/3  "<EM_Torque_Out_Nm>"
  Startup-Shutdown/3(Inverter_Status) -> Terminator/1
  Bus Creator/1 -> Inverter_Status/1  "Status"
  Subsystem/2(VSM) -> VSM/1, Bus Creator/5
  Faults/1 -> Bus Selector3/1
  Bus Selector3/1 -> Memory/1  "<RUN_Fault>"
  Bus Selector3/2 -> Memory2/1  "<ShutdownRequest>"
  Memory/1 -> Startup-Shutdown/5(RUN_Fault)
  Memory2/1 -> Startup-Shutdown/6(ShutdownRequest)

== system EcoSIM3_P2_C2_WIP/Powertrain/Electrical Storage System/ ESS Model/Plant/Electrical Plant Model ==
  P_in [W] : Inport
  Batt_Temp [C] : Inport  Port=2
  Current Calculation (Per Cell) : Subsystem
  Heat Calculation : Subsystem
  Memory1 : Memory  X0=300
  OCV Estimation : Subsystem
  "Resistance Estimation (Per Cell) " : Subsystem
  SOC Estimation (Per Cell) : Subsystem
  Terminal Voltage Calculation : Subsystem
  Batt_Current [A] : Outport
  Batt_SOC [%] : Outport  Port=2
  Batt_volt [V] : Outport  Port=3
  Batt_Heat [W] : Outport  Port=4
  Batt_volt_1 [V] : Outport  Port=5
  wires:
  P_in [W]/1 -> SOC Estimation (Per Cell)/1(P_in [W]), Current Calculation (Per Cell)/1(P_in [W])
  Terminal Voltage Calculation/1(Batt_Volt [V]) -> Batt_volt [V]/1, Memory1/1
  Current Calculation (Per Cell)/2(Cell_Current [A]) -> "Resistance Estimation (Per Cell) "/1(Cell_Current [A]), Heat Calculation/1(Cell_Current [A]), Terminal Voltage Calculation/3(Cell_Current [A]), OCV Estimation/2(Cell_Current [A])
  SOC Estimation (Per Cell)/1(SOC [%]) -> "Resistance Estimation (Per Cell) "/3(SOC [%]), Batt_SOC [%]/1, OCV Estimation/1(SOC [%])
  OCV Estimation/1(OCV [V]) -> Terminal Voltage Calculation/2(OCV [V])
  Current Calculation (Per Cell)/1(Batt_Current [A]) -> Batt_Current [A]/1
  Heat Calculation/1(Batt_Heat [W]) -> Batt_Heat [W]/1
  "Resistance Estimation (Per Cell) "/1(R_cell [Ohms]) -> Terminal Voltage Calculation/1(R_cell [Ohms]), Heat Calculation/2(R_cell [Ohms])
  Memory1/1 -> Batt_volt_1 [V]/1, Current Calculation (Per Cell)/2(Batt_volt [V])
  Batt_Temp [C]/1 -> "Resistance Estimation (Per Cell) "/2(Cell_Temp [C])

== system EcoSIM3_P2_C2_WIP/Powertrain/Electrical Storage System/ ESS Model/Plant/Power Calculation ==
  Input_Crnt [A] : Inport
  Batt_volt_1 [V] : Inport  Port=2
  Component_Power_Watts : Inport  Port=3
  Avg Power Calculation : Subsystem
  Integrator1 : Integrator
  P_in [W] : Outport
  Batt_Electrical_Energy : Outport  Port=2
  Batt_Electrical_Energy_Net : Outport  Port=3
  wires:
  Avg Power Calculation/1(P_in [W]) -> Batt_Electrical_Energy/1, Integrator1/1, P_in [W]/1  "Batt_Electrical_Energy"
  Input_Crnt [A]/1 -> Avg Power Calculation/1(Input_Crnt [A])
  Batt_volt_1 [V]/1 -> Avg Power Calculation/2(Batt_volt_1 [V])
  Integrator1/1 -> Batt_Electrical_Energy_Net/1  "Batt_Electrical_Energy_Net"
  Component_Power_Watts/1 -> Avg Power Calculation/3(Component_Power_Watts)

== system EcoSIM3_P2_C2_WIP/Powertrain/Electrical Storage System/ ESS Model/Plant/Thermal Model ==
  note: mC = 19395
  note: 1/7
  note: 273+30
  Batt_Heat [W] : Inport
  Bus Selector : BusSelector  OutputSignals=ESS_Thermal_Trigger
  Constant : Constant  Value=Plants.ESS.Mdl.Plant.Therm_Mdl.T_amb
  Constant5 : Constant  Value=273
  Convection_Multiplier : Constant  Value=0.4
  Divide : Product  Inputs=*/
  ESS_Over_Temp_Fault : Subsystem
  Fcn2 : Fcn  Expr=u/19395
  Fcn3 : Fcn  Expr=u/(193.52*19395)
  Gain : Gain
  Heat input for pack1 : Gain  Gain=1/Plants.ESS.Mdl.Plant.Therm_Mdl.M
  Integrator : Integrator  InitialConditionSource=external
  Normal : Constant
  Normal1 : Constant
  Product : Product  Inputs=**
  Subtract : Sum  Inputs=+-
  Subtract3 : Sum  Inputs=-+
  Subtract4 : Sum  Inputs=+-
  Switch : Switch  Criteria=u2 > Threshold  Threshold=0.5
  Switch1 : Switch  Criteria=u2 > Threshold  Threshold=0.5
  T_ambient : Constant  Value=Plants.ESS.Mdl.Plant.Therm_Mdl.T_amb
  Terminator : Terminator
  Terminator1 : Terminator
  fan_setting_HSC : Lookup_n-D  NumberOfTableDimensions=1  BreakpointsForDimension1=[35 45]  Table=[0 100]  ExtrapMethod=Clip  UseLastTableValue=on  InternalRulePriority=Speed  RndMeth=Simplest  InputSameDT=on
  heat_in_multiplier : Constant  Value=0.1
  heat_transfer_multiplier_coef : Lookup_n-D  NumberOfTableDimensions=1  BreakpointsForDimension1=[0 100]  Table=[0.05 1]  ExtrapMethod=Clip  UseLastTableValue=on  InternalRulePriority=Speed  RndMeth=Simplest  InputSameDT=on
  Batt_Temp [C] : Outport
  wires:
  Batt_Heat [W]/1 -> Heat input for pack1/1
  Integrator/1 -> Subtract/1, Subtract4/1  "T_B"
  Subtract3/1 -> Integrator/1  "T_B_dot"
  T_ambient/1 -> Subtract/2
  Subtract/1 -> Fcn3/1
  Fcn2/1 -> Subtract3/2  "heating"
  Constant/1 -> Integrator/2
  Constant5/1 -> Subtract4/2
  ESS_Over_Temp_Fault/1(Out1) -> Batt_Temp [C]/1  "Batt_Temp_C"
  Fcn3/1 -> Product/2
  Subtract4/1 -> fan_setting_HSC/1, ESS_Over_Temp_Fault/1(In1)  "Batt_Temp_C"
  Product/1 -> Subtract3/1  "cooling"
  Heat input for pack1/1 -> Divide/1, Gain/1
  Divide/1 -> Fcn2/1
  Switch1/1 -> Divide/2
  heat_transfer_multiplier_coef/1 -> Terminator1/1  "heat_transfer_multiplier"
  Gain/1 -> Terminator/1  "heat_in"
  fan_setting_HSC/1 -> heat_transfer_multiplier_coef/1  "fan_speed"
  Normal/1 -> Switch/3
  Normal1/1 -> Switch1/3
  heat_in_multiplier/1 -> Switch1/1
  Switch/1 -> Product/1
  [ESS_Over_temperature_Trigger] -> Bus Selector/1
  Bus Selector/1 -> Switch1/2, Switch/2  "<ESS_Thermal_Trigger>"
  Convection_Multiplier/1 -> Switch/1

== system EcoSIM3_P2_C2_WIP/Powertrain/Electrical Storage System/Soft ECU/Algorithm/A123 Documentation ==

== system EcoSIM3_P2_C2_WIP/Powertrain/Electrical Storage System/Soft ECU/Algorithm/Current Buffer ==
  Current : Inport
  Charge Buffer : Subsystem
  Current based EPO : Subsystem
  Discharge Buffer : Subsystem
  Terminator : Terminator
  charge buffer : Outport
  discharge buffer : Outport  Port=2
  wires:
  Current/1 -> Current based EPO/2(i_bat), Discharge Buffer/1(Current), Charge Buffer/1(Current)
  Discharge Buffer/1(Buffer) -> discharge buffer/1
  Charge Buffer/1(Buffer) -> charge buffer/1
  Discharge Buffer/2(dis_max) -> Current based EPO/1(dis_max)
  Current based EPO/1(epo_req) -> Terminator/1

== system EcoSIM3_P2_C2_WIP/Powertrain/Electrical Storage System/Soft ECU/Algorithm/Subsystem ==
  In1 : Inport
  In2 : Inport  Port=2
  In3 : Inport  Port=3
  In4 : Inport  Port=4
  In5 : Inport  Port=5
  In6 : Inport  Port=6
  In7 : Inport  Port=7
  In8 : Inport  Port=8
  In9 : Inport  Port=9
  In10 : Inport  Port=10
  Memory{,1..9} (10 alike) : Memory
  Out1 : Outport
  Out2 : Outport  Port=2
  Out3 : Outport  Port=3
  Out4 : Outport  Port=4
  Out5 : Outport  Port=5
  Out6 : Outport  Port=6
  Out7 : Outport  Port=7
  Out8 : Outport  Port=8
  Out9 : Outport  Port=9
  Out10 : Outport  Port=10
  wires:
  Memory3/1 -> Out4/1  "bcm_chgc_stat"
  Memory1/1 -> Out3/1  "bcm_mainc_stat"
  Memory2/1 -> Out5/1  "bcm_cpwr_cmd"
  Memory4/1 -> Out2/1  "bcm_hvil_mon"
  Memory5/1 -> Out6/1  "bcm_cpwr_mon"
  Memory/1 -> Out1/1  "bcm_ready"
  Memory6/1 -> Out7/1  "bcm_epo"
  In1/1 -> Memory/1
  In4/1 -> Memory3/1
  In7/1 -> Memory6/1
  In6/1 -> Memory5/1
  In5/1 -> Memory2/1
  In3/1 -> Memory1/1
  In2/1 -> Memory4/1
  Memory7/1 -> Out8/1  "bcm_veh_mon"
  In8/1 -> Memory7/1
  In9/1 -> Memory8/1
  Memory8/1 -> Out9/1  "chga_ena"
  In10/1 -> Memory9/1
  Memory9/1 -> Out10/1  "bcm_on_plug"

== system EcoSIM3_P2_C2_WIP/Powertrain/Engine/ Component Model/Sensors/Sensor lag ==
  i : Inport
  1st Order LPF of 1ms in Discrete Form : DiscreteTransferFcn  Numerator=[0.6321]  Denominator=[1 -0.3679]
  o : Outport
  wires:
  i/1 -> 1st Order LPF of 1ms in Discrete Form/1
  1st Order LPF of 1ms in Discrete Form/1 -> o/1

== system EcoSIM3_P2_C2_WIP/Powertrain/Engine/ Component Model/Sensors/Sensor lag1 ==
  i : Inport
  1st Order LPF of 1ms in Discrete Form : DiscreteTransferFcn  Numerator=[0.6321]  Denominator=[1 -0.3679]
  o : Outport
  wires:
  i/1 -> 1st Order LPF of 1ms in Discrete Form/1
  1st Order LPF of 1ms in Discrete Form/1 -> o/1

== system EcoSIM3_P2_C2_WIP/Powertrain/Engine/Soft ECU/Algorithm/TorqueRegulation ==
  Enigine_Speed : Inport
  Relay : Inport  Port=2
  Torque_Request : Inport  Port=3
  ISP_R : Inport  Port=4
  PCM_Wake : Inport  Port=5
  Compare To Constant : simulink/Logic and Bit Operations/Compare To Constant  relop===  const=3  OutDataTypeStr=boolean
  Compare To Constant1 : simulink/Logic and Bit Operations/Compare To Constant  relop===  const=2  OutDataTypeStr=boolean
  Compare To Constant2 : simulink/Logic and Bit Operations/Compare To Constant  relop===  const=4  OutDataTypeStr=boolean
  Constant : Constant  Value=0
  Enabled Subsystem : Subsystem  TreatAsAtomicUnit=on
  Enabled Subsystem1 : Subsystem  TreatAsAtomicUnit=on
  Enabled Subsystem2 : Subsystem  TreatAsAtomicUnit=on
  Engine_ : Constant  Value=Plants.ICE.Mdl.Plant.idle_w
  Engine_Red_Lining_Speed : Constant  Value=Plants.ICE.Mdl.Plant.red_line_w
  Enigine_Speed1 : InportShadow
  Multiport Switch : MultiPortSwitch  Inputs=4
  Subsystem : Subsystem
  Out1 : Outport
  wires:
  Compare To Constant1/1 -> Enabled Subsystem1/Enable
  Subsystem/2(Torque_Cmd) -> Enabled Subsystem2/1(Torque_Cmd_Nm)
  Compare To Constant2/1 -> Enabled Subsystem/Enable
  Compare To Constant/1 -> Enabled Subsystem2/Enable
  Enabled Subsystem1/1("Torque Command ") -> Multiport Switch/3
  Enabled Subsystem2/1("Torque Command ") -> Multiport Switch/4
  Multiport Switch/1 -> Out1/1
  Enabled Subsystem/1("Torque Command ") -> Multiport Switch/5
  Enigine_Speed/1 -> Enabled Subsystem2/2(Engine Speed [rad/s]), Enabled Subsystem1/2(Engine_Speed [rad/s]), Subsystem/1(Engine_Speed)
  Constant/1 -> Multiport Switch/2
  Engine_/1 -> Enabled Subsystem1/1(Idle_Speed)
  Engine_Red_Lining_Speed/1 -> Enabled Subsystem/1(Red_Line_Speed)
  Relay/1 -> Subsystem/2(ECM_Powerup)
  Torque_Request/1 -> Subsystem/3(Torque_Request)
  PCM_Wake/1 -> Subsystem/5(PCM_Wake)
  ISP_R/1 -> Subsystem/4(ISP_R)
  Subsystem/1(Mode) -> Compare To Constant/1, Compare To Constant2/1, Multiport Switch/1, Compare To Constant1/1
  Enigine_Speed1/1 -> Enabled Subsystem/2(Engine_Speed [rad/s])

== system EcoSIM3_P2_C2_WIP/Powertrain/Soft_ECUs_IO/From_Goto/Subsystem1/BAS_Relay ==
  In1 : Inport
  Constant6 : Constant
  Constant7 : Constant  Value=0
  Relay3 : Switch  Criteria=u2 > Threshold  Threshold=0.5
  Out1 : Outport
  wires:
  Constant6/1 -> Relay3/1
  Relay3/1 -> Out1/1  "BAS_Powerup"
  Constant7/1 -> Relay3/3
  In1/1 -> Relay3/2

== system EcoSIM3_P2_C2_WIP/Powertrain/Soft_ECUs_IO/From_Goto/Subsystem1/BMS Electrical ==
  In1 : Inport
  In2 : Inport  Port=2
  Constant : Constant
  Constant1 : Constant  Value=0
  Constant2 : Constant
  Constant3 : Constant  Value=0
  Relay : Switch  Criteria=u2 > Threshold  Threshold=0.5
  Relay1 : Switch  Criteria=u2 > Threshold  Threshold=0.5
  Out1 : Outport
  Out2 : Outport  Port=2
  wires:
  In1/1 -> Relay/2
  Constant/1 -> Relay/1
  Constant1/1 -> Relay/3
  Relay/1 -> Out1/1  "BMS_Powerup"
  Constant2/1 -> Relay1/1
  Constant3/1 -> Relay1/3
  In2/1 -> Relay1/2
  Relay1/1 -> Out2/1  "veh_wake"

== system EcoSIM3_P2_C2_WIP/Powertrain/Soft_ECUs_IO/From_Goto/Subsystem1/DCDC_Powerup ==
  In1 : Inport
  Constant2 : Constant
  Constant3 : Constant  Value=0
  Relay1 : Switch  Criteria=u2 > Threshold  Threshold=0.5
  Out1 : Outport
  wires:
  In1/1 -> Relay1/2
  Constant3/1 -> Relay1/3
  Constant2/1 -> Relay1/1
  Relay1/1 -> Out1/1  "DCDC_Powerup"

== system EcoSIM3_P2_C2_WIP/Powertrain/Soft_ECUs_IO/From_Goto/Subsystem1/EM_Relay ==
  In1 : Inport
  Constant2 : Constant
  Constant3 : Constant  Value=0
  Relay1 : Switch  Criteria=u2 > Threshold  Threshold=0.5
  Out1 : Outport
  wires:
  Relay1/1 -> Out1/1  "EM_Powerup"
  Constant2/1 -> Relay1/1
  Constant3/1 -> Relay1/3
  In1/1 -> Relay1/2
